simulink model "exe1"  (R2025b)
settings: Solver=VariableStepAuto  StartTime=0.0  StopTime=T_sim  RelTol=1e-3
values from neighbouring files (symbols this model uses):
  C1 = 1    [es310326.m]
  C2 = 1    [es310326.m]
  h1_ini = 0.7    [es310326.m]
  h2_ini = 0.6    [es310326.m]
  h2_ref = 1.2    [es310326.m]
  k = 0.05    [es310326.m]
  u1_ref = k*sqrt(h2_ref)    [es310326.m]
  u2_ref = u1_ref    [es310326.m]
libraries: cstblocks x1
settings Model: Creator=leonardoleggeri  LastModifiedBy=leonardoleggeri
settings DebuggingCC: UnderSpecifiedDimensionMsg=warning

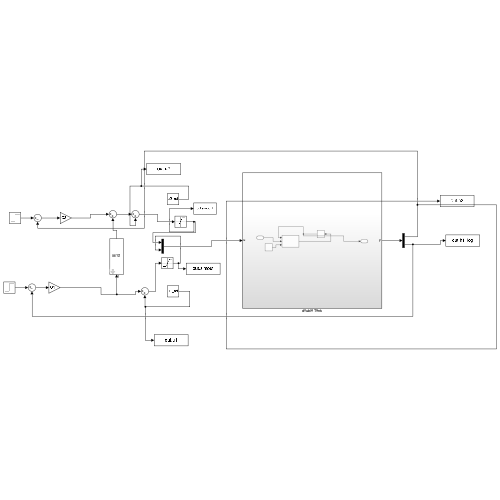
[thumbnail: Simulink's stored preview of the top-level diagram]
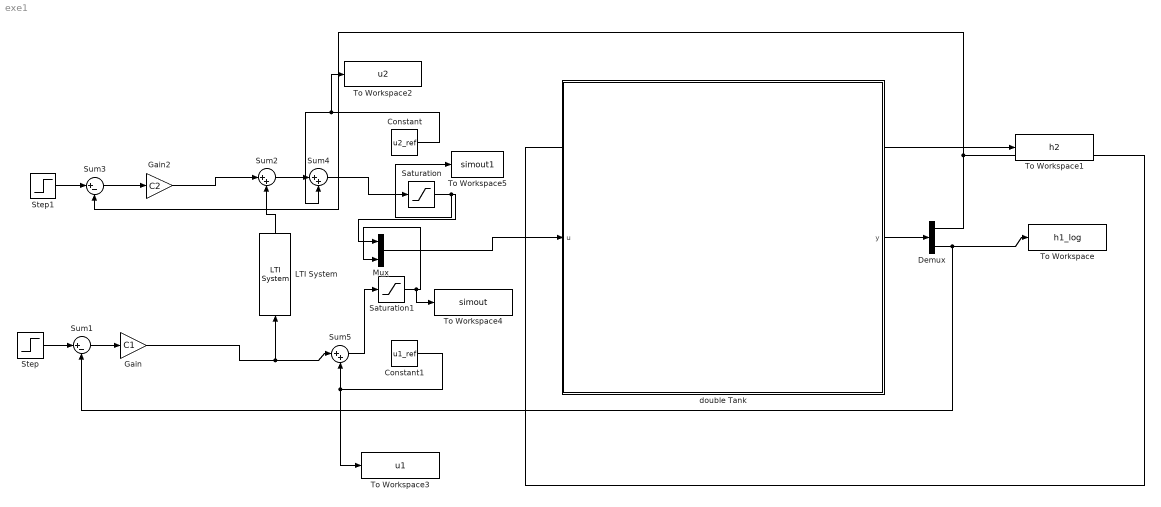
== system exe1 ==
  Constant : Constant  Value=u2_ref  VectorParams1D=off
  Constant1 : Constant  Value=u1_ref
  Demux : Demux  Outputs=2
  Gain : Gain  Gain=C1
  Gain2 : Gain  Gain=C2
  LTI System : cstblocks/LTI System  sys=M12  IC=[]  PadeOrder=0
  Mux : Mux  Inputs=2
  Saturation : Saturate
  Saturation1 : Saturate
  Step : Step  Before=h1_ini  After=h2_ref  SampleTime=0
  Step1 : Step  Before=h2_ini  After=h2_ref  SampleTime=0
  Sum1 : Sum  Inputs=|+-
  Sum2 : Sum  Inputs=|++
  Sum3 : Sum  Inputs=|+-
  Sum4 : Sum  Inputs=|++
  Sum5 : Sum  Inputs=|++
  To Workspace : ToWorkspace  VariableName=h1_log  SaveFormat=Timeseries  SampleTime=-1
  To Workspace1 : ToWorkspace  VariableName=h2  SaveFormat=Timeseries  SampleTime=-1
  To Workspace2 : ToWorkspace  VariableName=u2  SaveFormat=Timeseries  SampleTime=-1
  To Workspace3 : ToWorkspace  VariableName=u1  SaveFormat=Timeseries  SampleTime=-1
  To Workspace4 : ToWorkspace  VariableName=simout  SaveFormat=Timeseries  SampleTime=-1
  To Workspace5 : ToWorkspace  VariableName=simout1  SaveFormat=Timeseries  SampleTime=-1
  double Tank : Subsystem
  wires:
  Mux/1 -> double Tank/1(u)
  Step/1 -> Sum1/1
  Sum1/1 -> Gain/1
  Gain2/1 -> Sum2/1
  Sum3/1 -> Gain2/1
  Step1/1 -> Sum3/1
  Sum2/1 -> Sum4/1
  Sum4/1 -> Saturation/1
  Gain/1 -> Sum5/1, LTI System/1
  Sum5/1 -> Saturation1/1
  Constant1/1 -> To Workspace3/1, Sum5/2
  LTI System/1 -> Sum2/2
  double Tank/1(y) -> Demux/1
  Demux/1 -> To Workspace1/1, Sum3/2
  Demux/2 -> Sum1/2, To Workspace/1
  Constant/1 -> To Workspace2/1, Sum4/2
  Saturation/1 -> To Workspace5/1, Mux/1
  Saturation1/1 -> To Workspace4/1, Mux/2

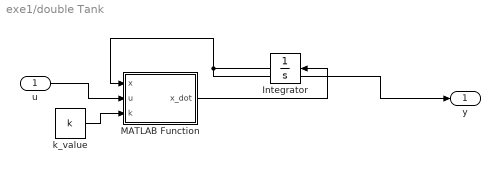
== system exe1/double Tank ==
  u : Inport
  Integrator : Integrator
  MATLAB Function : MATLAB Function  TreatAsAtomicUnit=on
  k_value : Constant  Value=k
  y : Outport
  wires:
  u/1 -> MATLAB Function/2(u)
  k_value/1 -> MATLAB Function/3(k)
  MATLAB Function/1(x_dot) -> Integrator/1
  Integrator/1 -> MATLAB Function/1(x), y/1

== matlab function exe1/double Tank/MATLAB Function ==
  data: x input; u input; x_dot output; k input
function x_dot= double_tank(x,u,k)
x_dot=zeroes(2,1);

x_dot(1)= u(1)-u(2);
x_dot(2)=u(2)-k*sqrt(x(2));

end
